simulink model "CSTD1_ClosedLoopLeadLag"  (R2020a)
settings: Solver=ode3  StartTime=0.0  StopTime=10  FixedStep=1e-3  MaxStep=1e-2  MinStep=1e-8  RelTol=1e-3  EnableMultiTasking=on
values from neighbouring files (symbols this model uses):
  dist_on = 1    [CSTD1_LeadLagDesign.m]
libraries: cstblocks x2, simulink x1
settings Model: Creator=am  LastModifiedBy=nwegy
settings DataIOCC: SaveFormat=Array  ReturnWorkspaceOutputs=off
settings OptimizationCC: LifeSpan=inf
settings DebuggingCC: UnderspecifiedInitializationDetection=Classic  MergeDetectMultiDrivingBlocksExec=none  SolverPrmCheckMsg=warning  StateNameClashWarn=warning  SFUnexpectedBacktrackingDiag=warning  SFNoUnconditionalDefaultTransitionDiag=warning  SFExecutionAtInitializationDiag=none  ArithmeticOperatorsInVariantConditions=warning
settings HardwareCC: ProdBitPerPointer=32  ProdBitPerSizeT=32  ProdBitPerPtrDiffT=32  ProdLargestAtomicFloat=None  ProdIntDivRoundTo=Undefined  ProdEndianess=Unspecified  ProdWordSize=32  ProdHWDeviceType=32-bit Generic
settings ModelReferenceCC: PropagateSignalLabelsOutOfModel=off
settings SFSimCC: SimUseLocalCustomCode=off  CustomCodeUndefinedFunction=UseInterfaceOnly
settings RTWCC: RTWUseLocalCustomCode=off
settings CodeAppCC: StateflowObjectComments=on
settings GRTTargetCC: TargetLangStandard=C89/C90 (ANSI)
settings ConfigComp: CovMetricSettings=dw  CovHtmlReporting=on  CovSaveCumulativeToWorkspaceVar=on  CovSaveSingleToWorkspaceVar=on  CovExternalEMLEnable=off  CovSFcnEnable=off

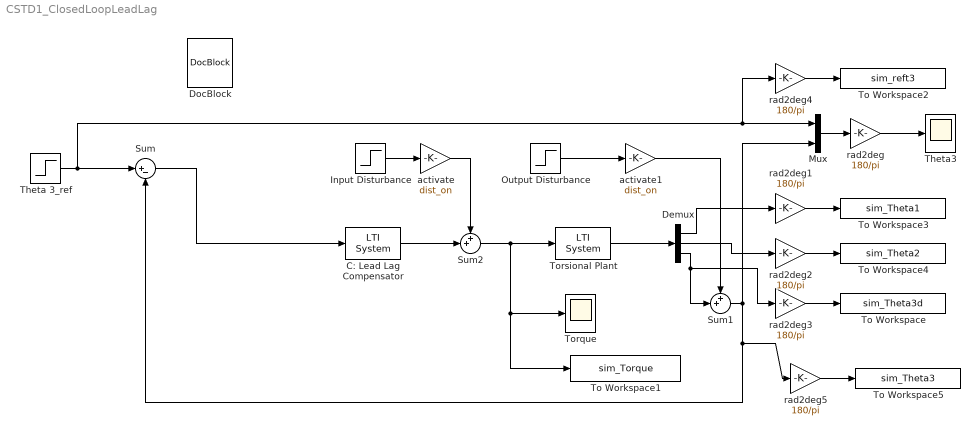
== system CSTD1_ClosedLoopLeadLag ==
  C: Lead Lag Compensator : cstblocks/LTI System  sys=C  IC=[]
  Demux : Demux  Outputs=3
  DocBlock : simulink/Model-Wide Utilities/DocBlock  DocumentType=Text
      content=|
      | % #########################################################################
      | % TUHH :: Institute for Control Systems :: Control Lab
      | % #########################################################################
      | % Experiment CSTD1: Control and Identification of a Torsional Plant
      | %
      | % Copyright Herbert Werner and Hamburg University of Technology, 2014
      | % #########################################################################
      | % This is the model containing the closed loop simulation for the lead lag
      | % compensator design.
      | %
      | % Further, the following variables need to be in the workspace to run the
      | % experiment:
      | %  - C       [tf or ss] : lead lag compensator
      | %  - sys     [tf or ss] : system
      | %  - dist_on [double]   : disturbance activation
      | %----------------------------
      | % v.1.0 - 15-11-2014
      | % by Antonio Mendez G
  Input Disturbance : Step  Time=7  After=0.2  SampleTime=0
  Mux : Mux  Inputs=2
  Output Disturbance : Step  Time=4  After=30*pi/180  SampleTime=0
  Sum : Sum  Inputs=|+-
  Sum1 : Sum  Inputs=++|
  Sum2 : Sum  Inputs=++|
  Theta 3_ref : Step  Time=0  After=2*pi  SampleTime=0
  Theta3 : Scope
  To Workspace : ToWorkspace  VariableName=sim_Theta3d  SampleTime=-1
  To Workspace1 : ToWorkspace  VariableName=sim_Torque  SampleTime=-1
  To Workspace2 : ToWorkspace  VariableName=sim_reft3  SampleTime=-1
  To Workspace3 : ToWorkspace  VariableName=sim_Theta1  SampleTime=-1
  To Workspace4 : ToWorkspace  VariableName=sim_Theta2  SampleTime=-1
  To Workspace5 : ToWorkspace  VariableName=sim_Theta3  SampleTime=-1
  Torque : Scope
  Torsional Plant : cstblocks/LTI System  sys=sys  IC=[]
  activate : Gain  Gain=dist_on
  activate1 : Gain  Gain=dist_on
  rad2deg{,1..5} (6 alike) : Gain  Gain=180/pi
  wires:
  Torsional Plant/1 -> Demux/1
  Sum/1 -> C: Lead Lag Compensator/1
  Demux/3 -> Sum1/2, rad2deg3/1
  Theta 3_ref/1 -> Sum/1, rad2deg4/1, Mux/1
  Mux/1 -> rad2deg/1
  rad2deg/1 -> Theta3/1
  Output Disturbance/1 -> activate1/1
  C: Lead Lag Compensator/1 -> Sum2/2
  Sum2/1 -> Torque/1, To Workspace1/1, Torsional Plant/1
  Input Disturbance/1 -> activate/1
  activate/1 -> Sum2/1
  activate1/1 -> Sum1/1
  Demux/1 -> rad2deg1/1
  Demux/2 -> rad2deg2/1
  rad2deg1/1 -> To Workspace3/1
  rad2deg2/1 -> To Workspace4/1
  rad2deg3/1 -> To Workspace/1
  rad2deg4/1 -> To Workspace2/1
  rad2deg5/1 -> To Workspace5/1
  Sum1/1 -> Mux/2, rad2deg5/1, Sum/2
